simulink model "projectSimulink"  (R2024b)
settings: Solver=VariableStepAuto  StartTime=0.0  StopTime=10.0  RelTol=1e-3
libraries: fuzblock x17
settings Model: Creator=ANA MARÍA  LastModifiedBy=ANA MARÍA

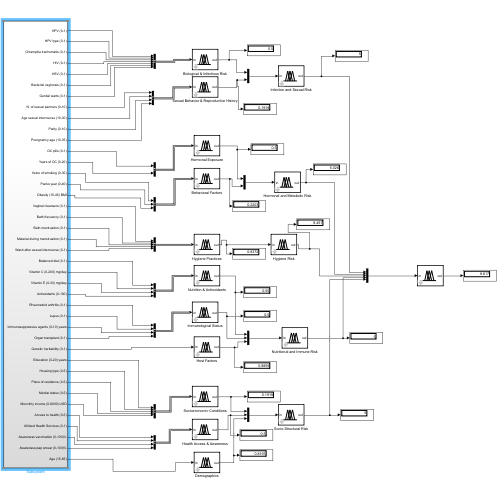
[thumbnail: Simulink's stored preview of the top-level diagram]
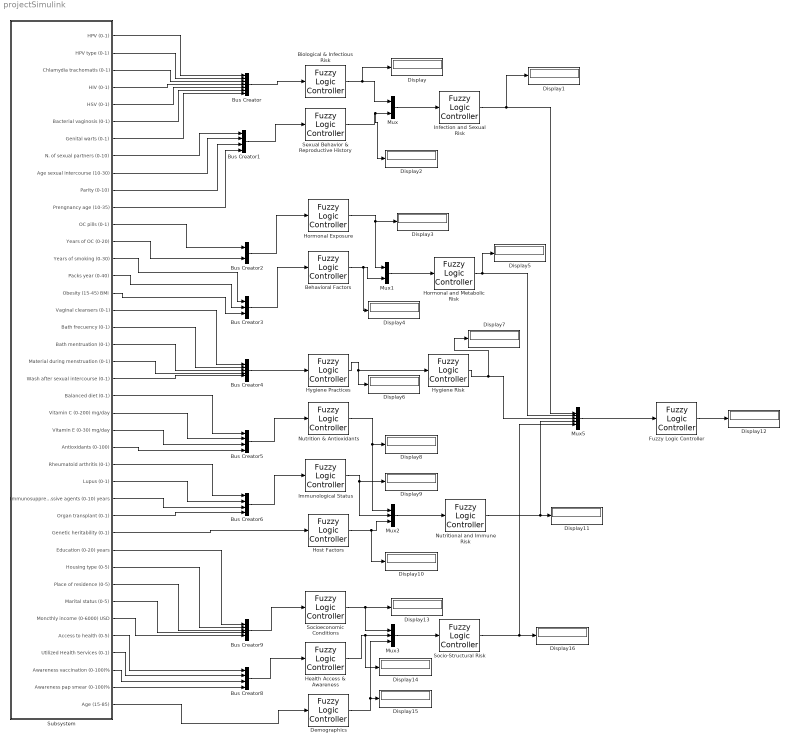
== system projectSimulink ==
  Behavioral Factors : fuzblock/Fuzzy Logic  Controller  FIS=fisBF  OutputSampleNumber=101  DataType=double  FuzzifiedInputs=off  RuleFiringStrengths=off  RuleOutputs=off  AggregatedOutputs=off  SimulateUsing=Interpreted execution  OutOfRangeInputValueMessage=warning  NoRuleFiredMessage=warning  EmptyOutputFuzzySetMessage=warning
  "Biological & Infectious Risk " : fuzblock/Fuzzy Logic  Controller  FIS=fisBIR  OutputSampleNumber=101  DataType=double  FuzzifiedInputs=off  RuleFiringStrengths=off  RuleOutputs=off  AggregatedOutputs=off  SimulateUsing=Interpreted execution  OutOfRangeInputValueMessage=warning  NoRuleFiredMessage=warning  EmptyOutputFuzzySetMessage=warning
  Bus Creator : BusCreator  Inputs=7
  Bus Creator{1,5..6,8} (4 alike) : BusCreator  Inputs=4
  Bus Creator2 : BusCreator  Inputs=2
  Bus Creator3 : BusCreator  Inputs=3
  Bus Creator4 : BusCreator  Inputs=5
  Bus Creator9 : BusCreator  Inputs=5
  Demographics : fuzblock/Fuzzy Logic  Controller  FIS=fisDF  OutputSampleNumber=101  DataType=double  FuzzifiedInputs=off  RuleFiringStrengths=off  RuleOutputs=off  AggregatedOutputs=off  SimulateUsing=Interpreted execution  OutOfRangeInputValueMessage=warning  NoRuleFiredMessage=warning  EmptyOutputFuzzySetMessage=warning
  Display{,1..16} (17 alike) : Display
  Fuzzy Logic Controller : fuzblock/Fuzzy Logic  Controller  FIS=fisCCR  OutputSampleNumber=101  DataType=double  FuzzifiedInputs=off  RuleFiringStrengths=off  RuleOutputs=off  AggregatedOutputs=off  SimulateUsing=Interpreted execution  OutOfRangeInputValueMessage=warning  NoRuleFiredMessage=warning  EmptyOutputFuzzySetMessage=warning
  Health Access & Awareness : fuzblock/Fuzzy Logic  Controller  FIS=fisHAA  OutputSampleNumber=101  DataType=double  FuzzifiedInputs=off  RuleFiringStrengths=off  RuleOutputs=off  AggregatedOutputs=off  SimulateUsing=Interpreted execution  OutOfRangeInputValueMessage=warning  NoRuleFiredMessage=warning  EmptyOutputFuzzySetMessage=warning
  Hormonal Exposure : fuzblock/Fuzzy Logic  Controller  FIS=fisHE  OutputSampleNumber=101  DataType=double  FuzzifiedInputs=off  RuleFiringStrengths=off  RuleOutputs=off  AggregatedOutputs=off  SimulateUsing=Interpreted execution  OutOfRangeInputValueMessage=warning  NoRuleFiredMessage=warning  EmptyOutputFuzzySetMessage=warning
  Hormonal and Metabolic Risk : fuzblock/Fuzzy Logic  Controller  FIS=fisHMRR  OutputSampleNumber=101  DataType=double  FuzzifiedInputs=off  RuleFiringStrengths=off  RuleOutputs=off  AggregatedOutputs=off  SimulateUsing=Interpreted execution  OutOfRangeInputValueMessage=warning  NoRuleFiredMessage=warning  EmptyOutputFuzzySetMessage=warning
  Host Factors : fuzblock/Fuzzy Logic  Controller  FIS=fisHF  OutputSampleNumber=101  DataType=double  FuzzifiedInputs=off  RuleFiringStrengths=off  RuleOutputs=off  AggregatedOutputs=off  SimulateUsing=Interpreted execution  OutOfRangeInputValueMessage=warning  NoRuleFiredMessage=warning  EmptyOutputFuzzySetMessage=warning
  Hygiene Practices : fuzblock/Fuzzy Logic  Controller  FIS=fisHP  OutputSampleNumber=101  DataType=double  FuzzifiedInputs=off  RuleFiringStrengths=off  RuleOutputs=off  AggregatedOutputs=off  SimulateUsing=Interpreted execution  OutOfRangeInputValueMessage=warning  NoRuleFiredMessage=warning  EmptyOutputFuzzySetMessage=warning
  Hygiene Risk : fuzblock/Fuzzy Logic  Controller  FIS=fisHR  OutputSampleNumber=101  DataType=double  FuzzifiedInputs=off  RuleFiringStrengths=off  RuleOutputs=off  AggregatedOutputs=off  SimulateUsing=Interpreted execution  OutOfRangeInputValueMessage=warning  NoRuleFiredMessage=warning  EmptyOutputFuzzySetMessage=warning
  Immunological Status : fuzblock/Fuzzy Logic  Controller  FIS=fisIS  OutputSampleNumber=101  DataType=double  FuzzifiedInputs=off  RuleFiringStrengths=off  RuleOutputs=off  AggregatedOutputs=off  SimulateUsing=Interpreted execution  OutOfRangeInputValueMessage=warning  NoRuleFiredMessage=warning  EmptyOutputFuzzySetMessage=warning
  "Infection and Sexual Risk " : fuzblock/Fuzzy Logic  Controller  FIS=fisIRR  OutputSampleNumber=101  DataType=double  FuzzifiedInputs=off  RuleFiringStrengths=off  RuleOutputs=off  AggregatedOutputs=off  SimulateUsing=Interpreted execution  OutOfRangeInputValueMessage=warning  NoRuleFiredMessage=warning  EmptyOutputFuzzySetMessage=warning
  Mux : Mux  Inputs=2
  Mux1 : Mux  Inputs=2
  Mux2 : Mux  Inputs=3
  Mux3 : Mux  Inputs=3
  Mux5 : Mux  Inputs=5
  Nutrition & Antioxidants : fuzblock/Fuzzy Logic  Controller  FIS=fisNAF  OutputSampleNumber=101  DataType=double  FuzzifiedInputs=off  RuleFiringStrengths=off  RuleOutputs=off  AggregatedOutputs=off  SimulateUsing=Interpreted execution  OutOfRangeInputValueMessage=warning  NoRuleFiredMessage=warning  EmptyOutputFuzzySetMessage=warning
  Nutritional and Immune Risk : fuzblock/Fuzzy Logic  Controller  FIS=fisNIR  OutputSampleNumber=101  DataType=double  FuzzifiedInputs=off  RuleFiringStrengths=off  RuleOutputs=off  AggregatedOutputs=off  SimulateUsing=Interpreted execution  OutOfRangeInputValueMessage=warning  NoRuleFiredMessage=warning  EmptyOutputFuzzySetMessage=warning
  "Sexual Behavior & Reproductive History " : fuzblock/Fuzzy Logic  Controller  FIS=fisSBRH  OutputSampleNumber=101  DataType=double  FuzzifiedInputs=off  RuleFiringStrengths=off  RuleOutputs=off  AggregatedOutputs=off  SimulateUsing=Interpreted execution  OutOfRangeInputValueMessage=warning  NoRuleFiredMessage=warning  EmptyOutputFuzzySetMessage=warning
  Socio-Structural Risk : fuzblock/Fuzzy Logic  Controller  FIS=fisSSRR  OutputSampleNumber=101  DataType=double  FuzzifiedInputs=off  RuleFiringStrengths=off  RuleOutputs=off  AggregatedOutputs=off  SimulateUsing=Interpreted execution  OutOfRangeInputValueMessage=warning  NoRuleFiredMessage=warning  EmptyOutputFuzzySetMessage=warning
  Socioeconomic Conditions : fuzblock/Fuzzy Logic  Controller  FIS=fisSEC  OutputSampleNumber=101  DataType=double  FuzzifiedInputs=off  RuleFiringStrengths=off  RuleOutputs=off  AggregatedOutputs=off  SimulateUsing=Interpreted execution  OutOfRangeInputValueMessage=warning  NoRuleFiredMessage=warning  EmptyOutputFuzzySetMessage=warning
  Subsystem : Subsystem
  wires:
  "Biological & Infectious Risk "/1 -> Display/1, Mux/1
  "Sexual Behavior & Reproductive History "/1 -> Display2/1, Mux/2
  Mux/1 -> "Infection and Sexual Risk "/1
  Mux1/1 -> Hormonal and Metabolic Risk/1
  Hormonal Exposure/1 -> Display3/1, Mux1/1
  Behavioral Factors/1 -> Display4/1, Mux1/2
  Hygiene Practices/1 -> Hygiene Risk/1, Display6/1
  Nutrition & Antioxidants/1 -> Display8/1, Mux2/1
  Immunological Status/1 -> Display9/1, Mux2/2
  Host Factors/1 -> Display10/1, Mux2/3
  Mux2/1 -> Nutritional and Immune Risk/1
  Socioeconomic Conditions/1 -> Display13/1, Mux3/1
  Health Access & Awareness/1 -> Display14/1, Mux3/2
  Demographics/1 -> Display15/1, Mux3/3
  Mux3/1 -> Socio-Structural Risk/1
  Mux5/1 -> Fuzzy Logic Controller/1
  "Infection and Sexual Risk "/1 -> Display1/1, Mux5/1
  Hormonal and Metabolic Risk/1 -> Display5/1, Mux5/2
  Hygiene Risk/1 -> Display7/1, Mux5/3
  Nutritional and Immune Risk/1 -> Display11/1, Mux5/4
  Socio-Structural Risk/1 -> Display16/1, Mux5/5
  Bus Creator/1 -> "Biological & Infectious Risk "/1
  Bus Creator1/1 -> "Sexual Behavior & Reproductive History "/1
  Bus Creator2/1 -> Hormonal Exposure/1
  Bus Creator3/1 -> Behavioral Factors/1
  Bus Creator4/1 -> Hygiene Practices/1
  Bus Creator5/1 -> Nutrition & Antioxidants/1
  Bus Creator6/1 -> Immunological Status/1
  Bus Creator8/1 -> Health Access & Awareness/1
  Bus Creator9/1 -> Socioeconomic Conditions/1
  Subsystem/1(HPV (0-1)) -> Bus Creator/1
  Subsystem/2(HPV type (0-1)) -> Bus Creator/2
  Subsystem/3(Chlamydia trachomatis (0-1)) -> Bus Creator/3
  Subsystem/4(HIV (0-1)) -> Bus Creator/4
  Subsystem/5(HSV (0-1)) -> Bus Creator/5
  Subsystem/6(Bacterial vaginosis (0-1)) -> Bus Creator/6
  Subsystem/7(Genital warts (0-1)) -> Bus Creator/7
  Subsystem/8(N. of sexual partners (0-10)) -> Bus Creator1/1
  Subsystem/9(Age sexual intercourse (10-30)) -> Bus Creator1/2
  Subsystem/10(Parity (0-10)) -> Bus Creator1/3
  Subsystem/11(Prengnancy age (10-35)) -> Bus Creator1/4
  Subsystem/12(OC pills (0-1)) -> Bus Creator2/1
  Subsystem/13(Years of OC (0-20)) -> Bus Creator2/2
  Subsystem/14(Years of smoking (0-30)) -> Bus Creator3/1
  Subsystem/15(Packs year (0-40)) -> Bus Creator3/2
  Subsystem/16(Obesity (15-45) BMI) -> Bus Creator3/3
  Subsystem/17(Vaginal cleansers (0-1)) -> Bus Creator4/1
  Subsystem/18(Bath frecuency (0-1)) -> Bus Creator4/2
  Subsystem/19(Bath mentruation (0-1)) -> Bus Creator4/3
  Subsystem/20(Material during menstruation (0-1)) -> Bus Creator4/4
  Subsystem/21(Wash after sexual intercourse (0-1)) -> Bus Creator4/5
  Subsystem/22(Balanced diet (0-1)) -> Bus Creator5/1
  Subsystem/23(Vitamin C (0-200) mg/day) -> Bus Creator5/2
  Subsystem/24(Vitamin E (0-30) mg/day) -> Bus Creator5/3
  Subsystem/25(Antioxidants (0-100)) -> Bus Creator5/4
  Subsystem/26(Rheumatoid arthritis (0-1)) -> Bus Creator6/1
  Subsystem/27(Lupus (0-1)) -> Bus Creator6/2
  Subsystem/28(Immunosuppressive agents (0-10) years) -> Bus Creator6/3
  Subsystem/29(Organ transplant (0-1)) -> Bus Creator6/4
  Subsystem/30(Genetic heritability (0-1)) -> Host Factors/1
  Subsystem/31(Education (0-20) years) -> Bus Creator9/1
  Subsystem/32(Housing type (0-5)) -> Bus Creator9/2
  Subsystem/33(Place of residence (0-5)) -> Bus Creator9/3
  Subsystem/34(Marital status (0-5)) -> Bus Creator9/4
  Subsystem/35(Moncthly income (0-6000) USD) -> Bus Creator9/5
  Subsystem/36(Access to health (0-5)) -> Bus Creator8/1
  Subsystem/37(Utilized Health Services (0-1)) -> Bus Creator8/2
  Subsystem/38(Awareness vaccination (0-100)%) -> Bus Creator8/3
  Subsystem/39(Awareness pap smear (0-100)%) -> Bus Creator8/4
  Subsystem/40(Age (15-85)) -> Demographics/1
  Fuzzy Logic Controller/1 -> Display12/1

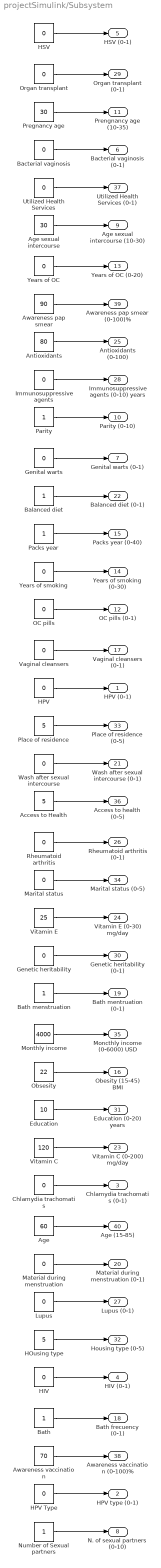
== system projectSimulink/Subsystem ==
  Access to Health : Constant  Value=5
  Age : Constant  Value=60
  Age sexual intercourse : Constant  Value=30
  Antioxidants : Constant  Value=80
  Awareness pap smear : Constant  Value=90
  Awareness vaccination : Constant  Value=70
  Bacterial vaginosis : Constant  Value=0
  Balanced diet : Constant
  Bath : Constant
  Bath menstruation : Constant
  Chlamydia trachomatis : Constant  Value=0
  Education : Constant  Value=10
  Genetic heritability : Constant  Value=0
  Genital warts : Constant  Value=0
  HIV : Constant  Value=0
  HOusing type : Constant  Value=5
  HPV : Constant  Value=0
  HPV Type : Constant  Value=0
  HSV : Constant  Value=0
  Immunosuppressive agents : Constant  Value=0
  Lupus : Constant  Value=0
  Marital status : Constant  Value=0
  Material during menstruation : Constant  Value=0
  Monthly income : Constant  Value=4000
  Number of Sexual partners : Constant
  OC pills : Constant  Value=0
  Obsesity : Constant  Value=22
  Organ transplant : Constant  Value=0
  Packs year : Constant
  Parity : Constant
  Place of residence : Constant  Value=5
  Pregnancy age : Constant  Value=30
  Rheumatoid arthritis : Constant  Value=0
  Utilized Health Services : Constant  Value=0
  Vaginal cleansers : Constant  Value=0
  Vitamin C : Constant  Value=120
  Vitamin E : Constant  Value=25
  Wash after sexual intercourse : Constant  Value=0
  Years of OC : Constant  Value=0
  Years of smoking : Constant  Value=0
  HPV (0-1) : Outport
  HPV type (0-1) : Outport  Port=2
  Chlamydia trachomatis (0-1) : Outport  Port=3
  HIV (0-1) : Outport  Port=4
  HSV (0-1) : Outport  Port=5
  Bacterial vaginosis (0-1) : Outport  Port=6
  Genital warts (0-1) : Outport  Port=7
  N. of sexual partners (0-10) : Outport  Port=8
  Age sexual intercourse (10-30) : Outport  Port=9
  Parity (0-10) : Outport  Port=10
  Prengnancy age (10-35) : Outport  Port=11
  OC pills (0-1) : Outport  Port=12
  Years of OC (0-20) : Outport  Port=13
  Years of smoking (0-30) : Outport  Port=14
  Packs year (0-40) : Outport  Port=15
  Obesity (15-45) BMI : Outport  Port=16
  Vaginal cleansers (0-1) : Outport  Port=17
  Bath frecuency (0-1) : Outport  Port=18
  Bath mentruation (0-1) : Outport  Port=19
  Material during menstruation (0-1) : Outport  Port=20
  Wash after sexual intercourse (0-1) : Outport  Port=21
  Balanced diet (0-1) : Outport  Port=22
  Vitamin C (0-200) mg/day : Outport  Port=23
  Vitamin E (0-30) mg/day : Outport  Port=24
  Antioxidants (0-100) : Outport  Port=25
  Rheumatoid arthritis (0-1) : Outport  Port=26
  Lupus (0-1) : Outport  Port=27
  Immunosuppressive agents (0-10) years : Outport  Port=28
  Organ transplant (0-1) : Outport  Port=29
  Genetic heritability (0-1) : Outport  Port=30
  Education (0-20) years : Outport  Port=31
  Housing type (0-5) : Outport  Port=32
  Place of residence (0-5) : Outport  Port=33
  Marital status (0-5) : Outport  Port=34
  Moncthly income (0-6000) USD : Outport  Port=35
  Access to health (0-5) : Outport  Port=36
  Utilized Health Services (0-1) : Outport  Port=37
  Awareness vaccination (0-100)% : Outport  Port=38
  Awareness pap smear (0-100)% : Outport  Port=39
  Age (15-85) : Outport  Port=40
  wires:
  Bath/1 -> Bath frecuency (0-1)/1
  Years of OC/1 -> Years of OC (0-20)/1
  Age/1 -> Age (15-85)/1
  Chlamydia trachomatis/1 -> Chlamydia trachomatis (0-1)/1
  Organ transplant/1 -> Organ transplant (0-1)/1
  HSV/1 -> HSV (0-1)/1
  Pregnancy age/1 -> Prengnancy age (10-35)/1
  Wash after sexual intercourse/1 -> Wash after sexual intercourse (0-1)/1
  Age sexual intercourse/1 -> Age sexual intercourse (10-30)/1
  Marital status/1 -> Marital status (0-5)/1
  Packs year/1 -> Packs year (0-40)/1
  Bacterial vaginosis/1 -> Bacterial vaginosis (0-1)/1
  Number of Sexual partners/1 -> N. of sexual partners (0-10)/1
  Utilized Health Services/1 -> Utilized Health Services (0-1)/1
  Vitamin C/1 -> Vitamin C (0-200) mg/day/1
  Awareness pap smear/1 -> Awareness pap smear (0-100)%/1
  Antioxidants/1 -> Antioxidants (0-100)/1
  Vaginal cleansers/1 -> Vaginal cleansers (0-1)/1
  Immunosuppressive agents/1 -> Immunosuppressive agents (0-10) years/1
  Parity/1 -> Parity (0-10)/1
  Genital warts/1 -> Genital warts (0-1)/1
  Balanced diet/1 -> Balanced diet (0-1)/1
  Years of smoking/1 -> Years of smoking (0-30)/1
  OC pills/1 -> OC pills (0-1)/1
  HPV/1 -> HPV (0-1)/1
  Material during menstruation/1 -> Material during menstruation (0-1)/1
  Place of residence/1 -> Place of residence (0-5)/1
  Access to Health/1 -> Access to health (0-5)/1
  Rheumatoid arthritis/1 -> Rheumatoid arthritis (0-1)/1
  Vitamin E/1 -> Vitamin E (0-30) mg/day/1
  Genetic heritability/1 -> Genetic heritability (0-1)/1
  Bath menstruation/1 -> Bath mentruation (0-1)/1
  HPV Type/1 -> HPV type (0-1)/1
  Monthly income/1 -> Moncthly income (0-6000) USD/1
  Obsesity/1 -> Obesity (15-45) BMI/1
  Education/1 -> Education (0-20) years/1
  Lupus/1 -> Lupus (0-1)/1
  HOusing type/1 -> Housing type (0-5)/1
  HIV/1 -> HIV (0-1)/1
  Awareness vaccination/1 -> Awareness vaccination (0-100)%/1
